simulink model "lab1_model_225"  (R2024b)
settings: Solver=ode45  StartTime=0.0  StopTime=sIn.simulation_time
undefined symbols (not defined in the file or in its folder): degs2rpm, drv, filt, gbox, mld, mot, rads2rpm, rpm2rads, sens, sIn, specs
libraries: simulink_extras x1
settings Model: Creator=bmm1  LastModifiedBy=ControlSystemsUser
settings SolverCC: ZeroCrossAlgorithm=Adaptive
settings DebuggingCC: IgnoredZcDiagnostic=none
settings RTWCC: GPUComputeCapability=3.5

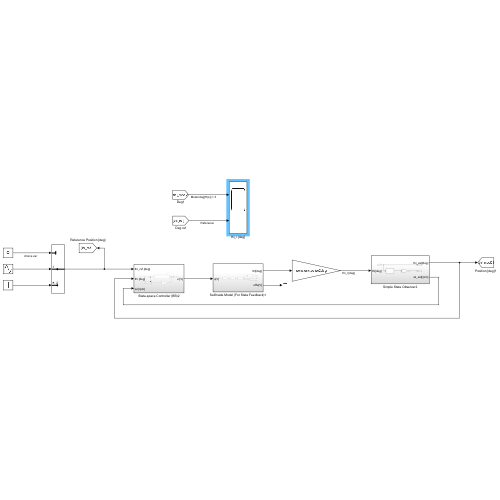
[thumbnail: Simulink's stored preview of the top-level diagram]
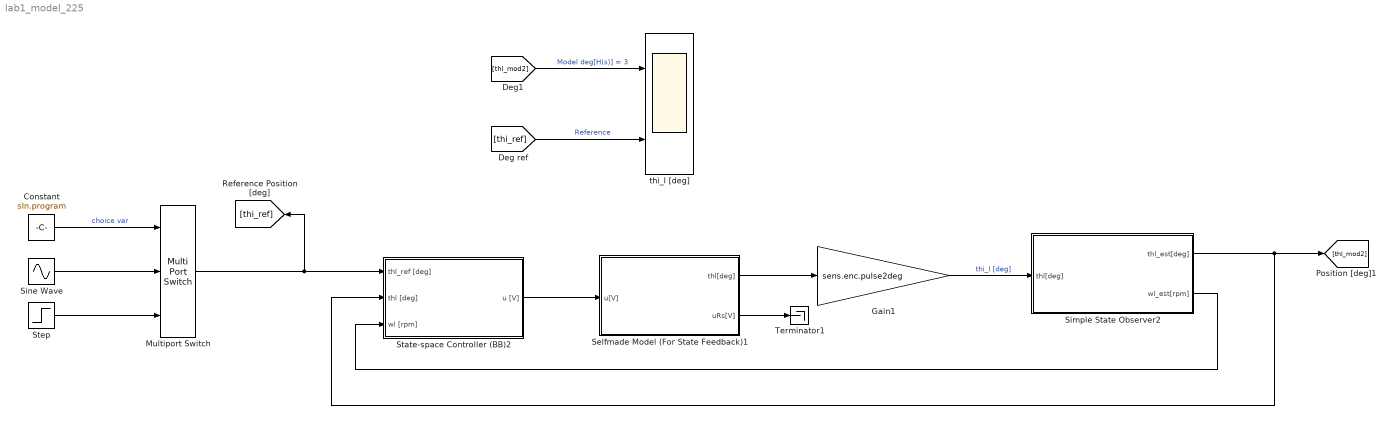
== system lab1_model_225 ==
  Constant : Constant  Value=sIn.program
  Gain1 : Gain  Gain=sens.enc.pulse2deg
  Multiport Switch : MultiPortSwitch  Inputs=2  SaturateOnIntegerOverflow=off  InputSameDT=off
  Selfmade Model (For State Feedback)1 : Subsystem
  Simple State Observer2 : Subsystem
  Sine Wave : Sin  Amplitude=sIn.Amp  Frequency=sIn.Freq  SampleTime=0
  State-space Controller (BB)2 : Subsystem
  Step : Step  Time=0  After=sIn.Amp  SampleTime=0
  Terminator1 : Terminator
  thi_l [deg] : Scope  NumInputPorts=2
  wires:
  [thi_ref] -> thi_l [deg]/2  "Reference"
  Sine Wave/1 -> Multiport Switch/2
  Step/1 -> Multiport Switch/3
  Constant/1 -> Multiport Switch/1  "choice var"
  Multiport Switch/1 -> State-space Controller (BB)2/1(thl_ref [deg]), [thi_ref]
  Simple State Observer2/2(wl_est[rpm]) -> State-space Controller (BB)2/3(wl [rpm])
  Simple State Observer2/1(thl_est[deg]) -> State-space Controller (BB)2/2(thl [deg]), [thl_mod2]
  Gain1/1 -> Simple State Observer2/1(thl[deg])  "thi_l [deg]"
  Selfmade Model (For State Feedback)1/2(uRs[V]) -> Terminator1/1
  State-space Controller (BB)2/1(u [V]) -> Selfmade Model (For State Feedback)1/1(u[V])
  Selfmade Model (For State Feedback)1/1(thl[deg]) -> Gain1/1
  [thl_mod2] -> thi_l [deg]/1  "Model deg[H(s)] = 3"

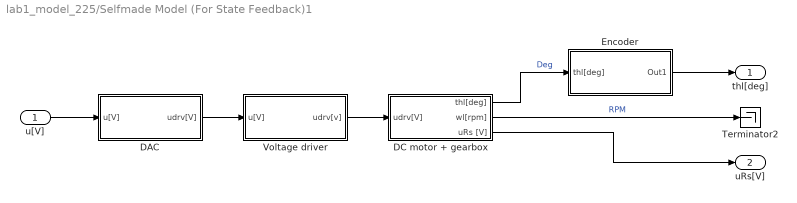
== system lab1_model_225/Selfmade Model (For State Feedback)1 ==
  u[V] : Inport
  DAC : Subsystem
  DC motor + gearbox : Subsystem
  Encoder : Subsystem
  Terminator2 : Terminator
  Voltage driver : Subsystem
  thl[deg] : Outport
  uRs[V] : Outport  Port=2
  wires:
  DC motor + gearbox/3(uRs [V]) -> uRs[V]/1
  Encoder/1(Out1) -> thl[deg]/1
  Voltage driver/1(udrv[v]) -> DC motor + gearbox/1(udrv[V])
  DAC/1(udrv[V]) -> Voltage driver/1(u[V])
  DC motor + gearbox/2(wl[rpm]) -> Terminator2/1  "RPM"
  u[V]/1 -> DAC/1(u[V])
  DC motor + gearbox/1(thl[deg]) -> Encoder/1(thl[deg])  "Deg"

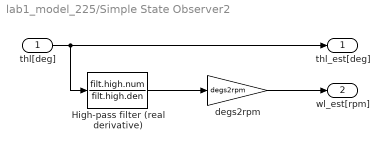
== system lab1_model_225/Simple State Observer2 ==
  thl[deg] : Inport
  High-pass filter (real derivative) : TransferFcn  Numerator=filt.high.num  Denominator=filt.high.den
  degs2rpm : Gain  Gain=degs2rpm
  thl_est[deg] : Outport
  wl_est[rpm] : Outport  Port=2
  wires:
  degs2rpm/1 -> wl_est[rpm]/1
  High-pass filter (real derivative)/1 -> degs2rpm/1
  thl[deg]/1 -> thl_est[deg]/1, High-pass filter (real derivative)/1

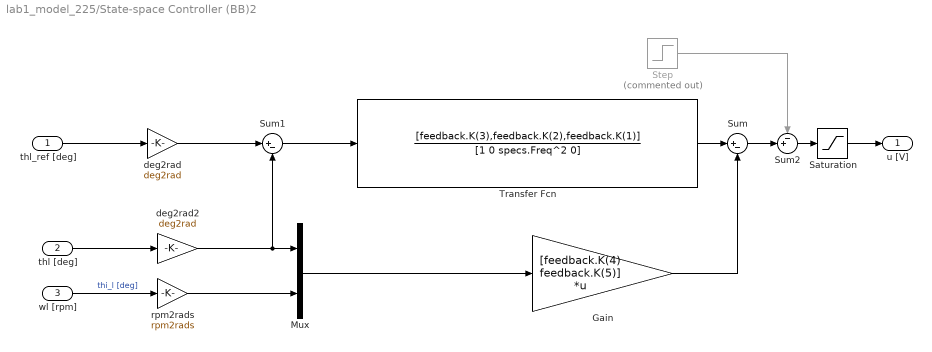
== system lab1_model_225/State-space Controller (BB)2 ==
  thl_ref [deg] : Inport
  thl [deg] : Inport  Port=2
  wl [rpm] : Inport  Port=3
  Gain : Gain  Gain=[feedback.K(4) feedback.K(5)]  Multiplication=Matrix(K*u)
  Mux : Mux  Inputs=2
  Saturation : Saturate  UpperLimit=10  LowerLimit=-10
  Step : Step  Commented=on  After=40  SampleTime=0
  Sum : Sum  Inputs=|+-
  Sum1 : Sum  Inputs=|+-
  Sum2 : Sum  Inputs=-+|
  Transfer Fcn : TransferFcn  Numerator=[feedback.K(3),feedback.K(2),feedback.K(1)]  Denominator=[1 0 specs.Freq^2 0]
  deg2rad : Gain  Gain=deg2rad
  deg2rad2 : Gain  Gain=deg2rad
  rpm2rads : Gain  Gain=rpm2rads
  u [V] : Outport
  wires:
  Step/1 -> Sum2/1
  Sum/1 -> Sum2/2
  Sum2/1 -> Saturation/1
  wl [rpm]/1 -> rpm2rads/1  "thi_l [deg]"
  Sum1/1 -> Transfer Fcn/1
  Gain/1 -> Sum/2
  rpm2rads/1 -> Mux/2
  Mux/1 -> Gain/1
  deg2rad/1 -> Sum1/1
  deg2rad2/1 -> Mux/1, Sum1/2
  thl [deg]/1 -> deg2rad2/1
  Saturation/1 -> u [V]/1
  Transfer Fcn/1 -> Sum/1
  thl_ref [deg]/1 -> deg2rad/1

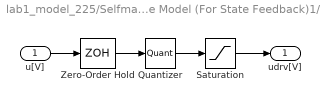
== system lab1_model_225/Selfmade Model (For State Feedback)1/DAC ==
  u[V] : Inport
  Quantizer : Quantizer  QuantizationInterval=daq.dac.q
  Saturation : Saturate  UpperLimit=10  LowerLimit=-10
  Zero-Order Hold : ZeroOrderHold  SampleTime=1e-3
  udrv[V] : Outport
  wires:
  Saturation/1 -> udrv[V]/1
  Quantizer/1 -> Saturation/1
  u[V]/1 -> Zero-Order Hold/1
  Zero-Order Hold/1 -> Quantizer/1

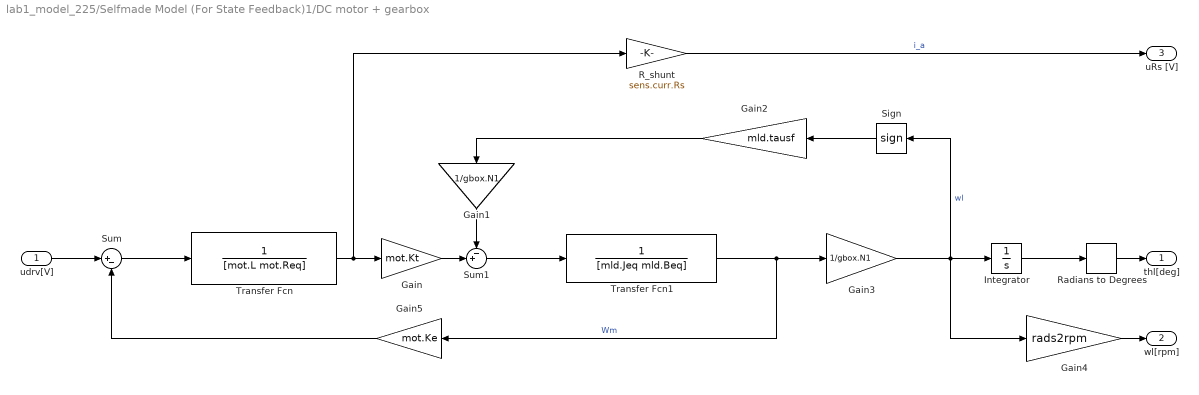
== system lab1_model_225/Selfmade Model (For State Feedback)1/DC motor + gearbox ==
  udrv[V] : Inport
  Gain : Gain  Gain=mot.Kt
  Gain1 : Gain  Gain=1/gbox.N1
  Gain2 : Gain  Gain=mld.tausf
  Gain3 : Gain  Gain=1/gbox.N1
  Gain4 : Gain  Gain=rads2rpm
  Gain5 : Gain  Gain=mot.Ke
  Integrator : Integrator
  R_shunt : Gain  Gain=sens.curr.Rs
  Radians to Degrees : simulink_extras/Transformations/Radians to Degrees
  Sign : Signum  ZeroCross=off
  Sum : Sum  Inputs=|+-
  Sum1 : Sum  Inputs=-+|
  Transfer Fcn : TransferFcn  Denominator=[mot.L mot.Req]
  Transfer Fcn1 : TransferFcn  Denominator=[mld.Jeq mld.Beq]
  thl[deg] : Outport
  wl[rpm] : Outport  Port=2
  uRs [V] : Outport  Port=3
  wires:
  R_shunt/1 -> uRs [V]/1  "i_a"
  Gain5/1 -> Sum/2
  Gain/1 -> Sum1/2
  Sum1/1 -> Transfer Fcn1/1
  Gain4/1 -> wl[rpm]/1
  Radians to Degrees/1 -> thl[deg]/1
  Integrator/1 -> Radians to Degrees/1
  Gain3/1 -> Integrator/1, Sign/1, Gain4/1  "wl"
  Transfer Fcn1/1 -> Gain3/1, Gain5/1  "Wm"
  Sign/1 -> Gain2/1
  Gain2/1 -> Gain1/1
  Gain1/1 -> Sum1/1
  Transfer Fcn/1 -> Gain/1, R_shunt/1
  Sum/1 -> Transfer Fcn/1
  udrv[V]/1 -> Sum/1

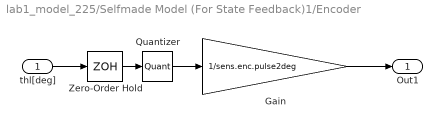
== system lab1_model_225/Selfmade Model (For State Feedback)1/Encoder ==
  thl[deg] : Inport
  Gain : Gain  Gain=1/sens.enc.pulse2deg
  Quantizer : Quantizer  QuantizationInterval=sens.enc.pulse2deg
  Zero-Order Hold : ZeroOrderHold  SampleTime=1e-3
  Out1 : Outport
  wires:
  Zero-Order Hold/1 -> Quantizer/1
  Quantizer/1 -> Gain/1
  Gain/1 -> Out1/1
  thl[deg]/1 -> Zero-Order Hold/1

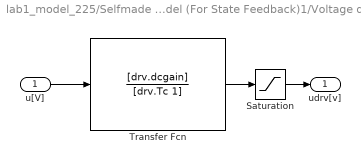
== system lab1_model_225/Selfmade Model (For State Feedback)1/Voltage driver ==
  u[V] : Inport
  Saturation : Saturate  UpperLimit=12  LowerLimit=-12
  Transfer Fcn : TransferFcn  Numerator=[drv.dcgain]  Denominator=[drv.Tc 1]
  udrv[v] : Outport
  wires:
  Saturation/1 -> udrv[v]/1
  Transfer Fcn/1 -> Saturation/1
  u[V]/1 -> Transfer Fcn/1
